simulink model "verify_Display_THB6_mdl"  (R2016b)
settings: Solver=VariableStepDiscrete  StartTime=0  StopTime=1  MaxStep=1  RelTol=1e-3  EnableMultiTasking=on
libraries: carnot x7
settings Model: Creator=drhf  LastModifiedBy=User
settings DataIOCC: SaveFormat=Array  SignalLoggingSaveFormat=ModelDataLogs
settings OptimizationCC: ExpressionDepthLimit=2147483647  LifeSpan=inf
settings DebuggingCC: UnderspecifiedInitializationDetection=Classic  MergeDetectMultiDrivingBlocksExec=none  SolverPrmCheckMsg=warning  FcnCallInpInsideContextMsg=warning  StateNameClashWarn=warning  SFUnexpectedBacktrackingDiag=warning  SFNoUnconditionalDefaultTransitionDiag=warning  SFExecutionAtInitializationDiag=none
settings HardwareCC: ProdBitPerPointer=32  ProdBitPerSizeT=32  ProdBitPerPtrDiffT=32  ProdLargestAtomicFloat=None  ProdIntDivRoundTo=Undefined  ProdEndianess=Unspecified  ProdWordSize=32  ProdHWDeviceType=32-bit Generic
settings ModelReferenceCC: PropagateSignalLabelsOutOfModel=off
settings GRTTargetCC: TargetLangStandard=C89/C90 (ANSI)  GeneratePreprocessorConditionals=Disable all  CombineOutputUpdateFcns=off  GRTInterface=on
settings ConfigComp: CovMetricSettings=dw  CovHtmlReporting=on  CovSaveCumulativeToWorkspaceVar=on  CovSaveSingleToWorkspaceVar=on  CovExternalEMLEnable=off

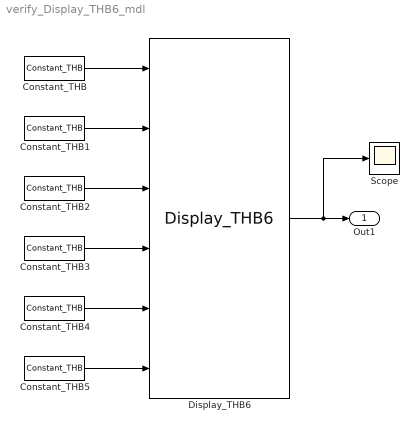
== system verify_Display_THB6_mdl ==
  Constant_THB : carnot/Source/Simple/Constant_THB  t=40  mdot=600/3600  p=1e5  mID=No Pressure Drop  fluid=Water  mix=0  mix2=0  mix3=0  dia=0.02  hgt=0
  Constant_THB1 : carnot/Source/Simple/Constant_THB  t=40  mdot=600/3600  p=5e5  mID=No Pressure Drop  fluid=Water  mix=0  mix2=0  mix3=0  dia=0.02  hgt=0
  Constant_THB2 : carnot/Source/Simple/Constant_THB  t=40  mdot=600/3600  p=3e5  mID=No Pressure Drop  fluid=Water  mix=0  mix2=0  mix3=0  dia=0.02  hgt=0
  Constant_THB3 : carnot/Source/Simple/Constant_THB  t=40  mdot=600/3600  p=6e5  mID=No Pressure Drop  fluid=Water  mix=0  mix2=0  mix3=0  dia=0.02  hgt=0
  Constant_THB4 : carnot/Source/Simple/Constant_THB  t=40  mdot=600/3600  p=4e5  mID=No Pressure Drop  fluid=Water  mix=0  mix2=0  mix3=0  dia=0.02  hgt=0
  Constant_THB5 : carnot/Source/Simple/Constant_THB  t=40  mdot=600/3600  p=2e5  mID=No Pressure Drop  fluid=Water  mix=0  mix2=0  mix3=0  dia=0.02  hgt=0
  Display_THB6 : carnot/Outputs/Display_THB6  t=off  m=off  p=on  id=off  mix=off  d=off
  Scope : Scope
  Out1 : Outport
  wires:
  Display_THB6/1 -> Scope/1, Out1/1
  Constant_THB/1 -> Display_THB6/1
  Constant_THB1/1 -> Display_THB6/2
  Constant_THB2/1 -> Display_THB6/3
  Constant_THB3/1 -> Display_THB6/4
  Constant_THB4/1 -> Display_THB6/5
  Constant_THB5/1 -> Display_THB6/6
